simulink model "NonLinearModel"  (R2018a)
settings: Solver=VariableStepAuto  StartTime=0.0  StopTime=10  RelTol=1e-3
undefined symbols (not defined in the file): netThrust, tspan, x0
libraries: simulink x3, dspindex x3
settings Model: Creator=ojack123  LastModifiedBy=ojack123
settings OptimizationCC: DefaultParameterBehavior=Inlined  BufferReuse=off
settings DebuggingCC: InitInArrayFormatMsg=none

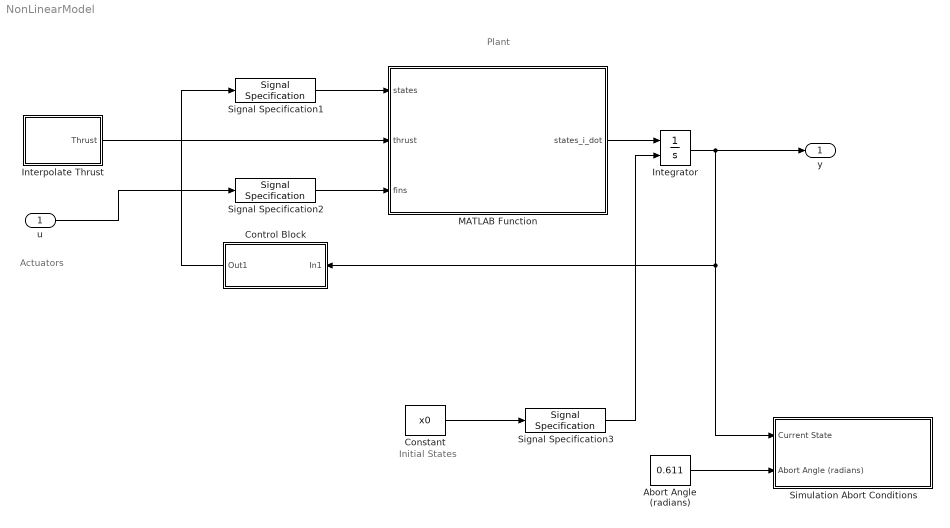
== system NonLinearModel ==
  note: Actuators
  note: Plant
  note: Initial States
  u : Inport
  Abort Angle (radians) : Constant  Value=0.611
  Constant : Constant  Value=x0
  Control Block : Subsystem
  Integrator : Integrator  InitialConditionSource=external  InitialCondition="[0 0 0 0 0 0.5 0 0    0.049979      0.99875 0.0 0.0 0]"
  Interpolate Thrust : Subsystem
  MATLAB Function : MATLAB Function  TreatAsAtomicUnit=on
  Signal Specification1 : SignalSpecification  Dimensions=[13 1]
  Signal Specification2 : SignalSpecification  Dimensions=[4 1]
  Signal Specification3 : SignalSpecification  Dimensions=[13 1]
  Simulation Abort Conditions : Subsystem
  y : Outport
  wires:
  MATLAB Function/1(states_i_dot) -> Integrator/1
  Interpolate Thrust/1(Thrust) -> MATLAB Function/2(thrust)
  Constant/1 -> Signal Specification3/1
  Integrator/1 -> y/1, Control Block/1(In1), Simulation Abort Conditions/1(Current State)
  Abort Angle (radians)/1 -> Simulation Abort Conditions/2(Abort Angle (radians))
  u/1 -> Signal Specification2/1
  Signal Specification1/1 -> MATLAB Function/1(states)
  Signal Specification2/1 -> MATLAB Function/3(fins)
  Signal Specification3/1 -> Integrator/2
  Control Block/1(Out1) -> Signal Specification1/1

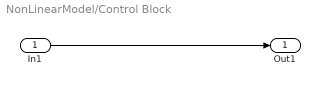
== system NonLinearModel/Control Block ==
  In1 : Inport
  Out1 : Outport
  wires:
  In1/1 -> Out1/1

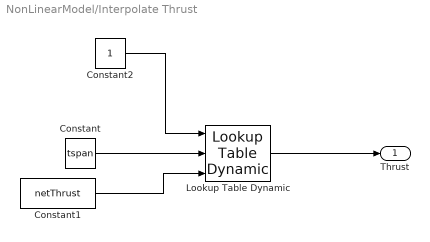
== system NonLinearModel/Interpolate Thrust ==
  Constant : Constant  Value=tspan  VectorParams1D=off
  Constant1 : Constant  Value=netThrust  VectorParams1D=off
  Constant2 : Constant
  Lookup Table Dynamic : simulink/Lookup Tables/Lookup Table Dynamic  LookUpMeth=Interpolation-Use End Values  OutDataType=fixdt('double')  OutScaling=2^-10  OutDataTypeStr=Inherit: Inherit via back propagation  RndMeth=Nearest  DoSatur=off
      settings: SourceProductName=Simulink
  Thrust : Outport
  wires:
  Constant2/1 -> Lookup Table Dynamic/1
  Lookup Table Dynamic/1 -> Thrust/1
  Constant/1 -> Lookup Table Dynamic/2
  Constant1/1 -> Lookup Table Dynamic/3

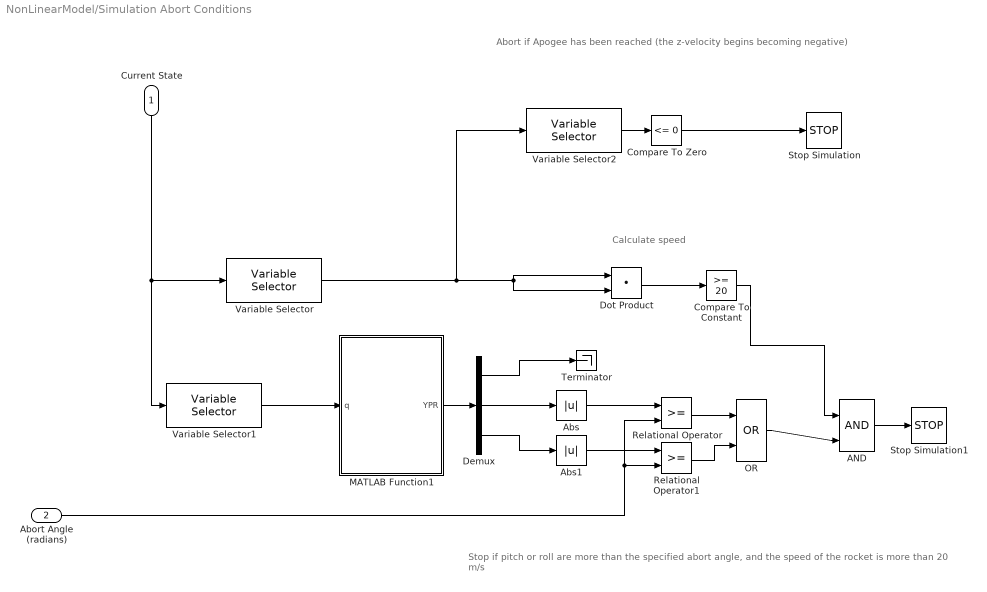
== system NonLinearModel/Simulation Abort Conditions ==
  note: Stop if pitch or roll are more than the specified abort angle, and the speed of the rocket is more than 20 m/s
  note: Calculate speed
  note: Abort if Apogee has been reached (the z-velocity begins becoming negative)
  Current State : Inport
  Abort Angle (radians) : Inport  Port=2
  AND : Logic  IconShape=distinctive  AllPortsSameDT=off  OutDataTypeStr=boolean
  Abs : Abs
  Abs1 : Abs
  Compare To Constant : simulink/Logic and Bit Operations/Compare To Constant  relop=>=  const=20  OutDataTypeStr=boolean
  Compare To Zero : simulink/Logic and Bit Operations/Compare To Zero  relop=<=  OutDataTypeStr=boolean
  Demux : Demux  Outputs=3
  Dot Product : DotProduct  InputSameDT=on  OutDataTypeStr=Inherit: Inherit via internal rule
  MATLAB Function1 : MATLAB Function  TreatAsAtomicUnit=on
  OR : Logic  Operator=OR  IconShape=distinctive  AllPortsSameDT=off  OutDataTypeStr=boolean
  Relational Operator : RelationalOperator  OutDataTypeStr=boolean  RndMeth=Simplest
  Relational Operator1 : RelationalOperator  OutDataTypeStr=boolean  RndMeth=Simplest
  Stop Simulation : Stop
  Stop Simulation1 : Stop
  Terminator : Terminator
  Variable Selector : dspindex/Variable Selector  NumInputs=1  rowsOrCols=Rows  IdxMode=Fixed  Elements=[4 5 6]  ZerOneIdxMode=One-based  errmode=Clip Index  FillMode=on  FillValues=0
  Variable Selector1 : dspindex/Variable Selector  NumInputs=1  rowsOrCols=Rows  IdxMode=Fixed  Elements=[7 8 9 10]  ZerOneIdxMode=One-based  errmode=Clip Index  FillMode=on  FillValues=0
  Variable Selector2 : dspindex/Variable Selector  NumInputs=1  rowsOrCols=Rows  IdxMode=Fixed  Elements=3  ZerOneIdxMode=One-based  errmode=Clip Index  FillMode=on  FillValues=0
  wires:
  Variable Selector/1 -> Dot Product/1, Dot Product/2, Variable Selector2/1
  OR/1 -> AND/2
  Compare To Zero/1 -> Stop Simulation/1
  Current State/1 -> Variable Selector/1, Variable Selector1/1
  Relational Operator/1 -> OR/1
  Relational Operator1/1 -> OR/2
  Variable Selector2/1 -> Compare To Zero/1
  Abort Angle (radians)/1 -> Relational Operator/2, Relational Operator1/2
  Abs1/1 -> Relational Operator1/1
  Abs/1 -> Relational Operator/1
  Compare To Constant/1 -> AND/1
  AND/1 -> Stop Simulation1/1
  Dot Product/1 -> Compare To Constant/1
  Variable Selector1/1 -> MATLAB Function1/1(q)
  Demux/2 -> Abs/1
  Demux/3 -> Abs1/1
  Demux/1 -> Terminator/1
  MATLAB Function1/1(YPR) -> Demux/1

== matlab function NonLinearModel/Simulation Abort Conditions/MATLAB Function1 ==
  data: q input; YPR output
function YPR = euler_from_q(q)
y = 0;
p = 0;
r = 0;
YPR = dcm_to_euler(dcm_from_q(q));

end
% ~~~~~~~~~~~~~~~~~~~~~~~~~~~~~~~~~~~~~~~~~~~~~~
function Q = dcm_from_q(q)
% ~~~~~~~~~~~~~~~~~~~~~~~
%{
  This function calculates the direction cosine matrix
  from the quaternion.

  q - quaternion (where q(4) is the scalar part)
  Q - direction cosine matrix
%}
% ----------------------------------------------
Q  = zeros(3);
q1 = 0;
q2 = 0;
q3 = 0;
q4 = 0;
q1 = q(1); q2 = q(2); q3 = q(3); q4 = q(4);

Q = [q1^2-q2^2-q3^2+q4^2,      2*(q1*q2+q3*q4),       2*(q1*q3-q2*q4);
         2*(q1*q2-q3*q4), -q1^2+q2^2-q3^2+q4^2,       2*(q2*q3+q1*q4);
         2*(q1*q3+q2*q4),      2*(q2*q3-q1*q4),  -q1^2-q2^2+q3^2+q4^2 ];
end %dcm_from_q
% ~~~~~~~~~~~~~~~~~~~~~~~~~~~~~~~~~~~~~~~~~~~~~~

% ~~~~~~~~~~~~~~~~~~~~~~~~~~~~~~~~~~~~~~~~~~~~~~~
function ABG = dcm_to_euler(Q)
% ~~~~~~~~~~~~~~~~~~~~~~~~~~~~~~~~~~~~~~~~~~~
%{
  This function finds the angles of the classical Euler sequence
  R3(gamma)*R1(beta)*R3(alpha) from the direction cosine matrix

  Q     - direction cosine matrix
  alpha - first angle of the sequence (deg)
  beta  - second angle of the sequence (deg)
  gamma - third angle of the sequence (deg)

  User M-function required: atan2d_0_360
%}
% -----------------------------------------------
alpha = 0;
beta  = 0;
gamma = 0;
alpha = atan2_0_360(Q(3,1), -Q(3,2));
beta  = acos(Q(3,3));
gamma = atan2_0_360(Q(1,3), Q(2,3));
ABG = [alpha beta gamma];

end
% ~~~~~~~~~~~~~~~~~~~~~~~~~~~~~~~~~~~~~~~~~~~~~~~


% ~~~~~~~~~~~~~~~~~~~~~~~~~~~~~~~~~~~~~~~~~~~~~~
function out = atan2_0_360(y,x)
% ~~~~~~~~~~~~~~~~~~~~~~~~~~~~
%{
  This function calculates the arc tangent of y/x in degrees
  and places the result in the range [0, 360].

  t - angle in degrees

%}
% ----------------------------------------------
y = 0;
x = 0;
t = 0;
out = 0;
y = rad2deg(y);
x = rad2deg(x);

if x == 0
    if y == 0
        t = 0;
    elseif y > 0
        t = 90;
    else
        t = 270;
    end    
elseif x > 0
    if y >= 0
        t = atand(y/x);
    else
        t = atand(y/x) + 360;
    end    
elseif x < 0   
    if y == 0
        t = 180;
    else
        t = atand(y/x) + 180;
    end       
end
out = deg2rad(t);
end

% ~~~~~~~~~~~~~~~~~~~~~~~~~~~~~~~~~~~~~~~~~~~~~~

== matlab function NonLinearModel/MATLAB Function ==
  data: states input; states_i_dot output; thrust input; fins input
function states_i_dot = EquationsOfMotion(states,thrust,fins)
   rocketStruct = load('rocket');
%% Define the quaternions 
    q           = states(7:10);
%% External Forces (inertial frame)
% Aerodynamic forces due to rocket body
    vel_i       = states(4:6);
    vel_b       = quaternion_I_to_B(q,vel_i);
    speed       = norm(vel_i);
    alpha       = atan2(vel_b(1),vel_b(3));
    beta        = asin(vel_b(2)/speed);
    Cx_v        = rocketStruct.rocket.Cla * (alpha);
    Cy_v        = rocketStruct.rocket.Clb * (beta);
    Cz_v        = 0.05*rocketStruct.rocket.Cd0; % Estimating the drag to be directly opposite the nose
    C_v         = [-Cx_v; -Cy_v; -Cz_v];
    Fad_v       = 0.5*(1.225)*rocketStruct.rocket.area*(speed^2).*C_v;
    Rvel2body   = (R2(-alpha)*R3(beta))';
    Fad_b       = Rvel2body *Fad_v;
Fad_i       = quaternion_B_to_I(q,Fad_b);
    
Fg_i        = [0;0;-9.8*rocketStruct.rocket.m];
    
Fexternal_i = Fg_i +Fad_i;
%% Thrust force
   thrust_b = [0;0;thrust];
netThrust_i = quaternion_B_to_I(q,thrust_b); 
    
%% Net Force on the rocket body
Fnet_i      = Fexternal_i + netThrust_i;

%% External Moments (inertial frame)
% Rotate the distance from CP to CG into the inertial frame
    cp2cg_b     = rocketStruct.rocket.dcg-rocketStruct.rocket.dcp;
    cp2cg_i     = quaternion_B_to_I(q,cp2cg_b); % distance from the cp to cg in inertial frame
% Moment due to aerodynamic force of rocket body
Mad_i       = cross(cp2cg_i,Fad_i);
% Net External Moments
Mexternal_i = Mad_i;
    
%% Moments due to Fins
% Fin locations (body fixed)
    finLatOffset = 0.1; % Flipper offset from z-axis
    finCGOffset  = -rocketStruct.rocket.dcg(3); % Flipper offset from the CG
    r1_b         = [finLatOffset;  0;            finCGOffset];
    r2_b         = [0;             finLatOffset; finCGOffset];
    r3_b         = [-finLatOffset; 0;            finCGOffset];
    r4_b         = [0;            -finLatOffset; finCGOffset];
% Fin forces
    F1_b         = [0       ; fins(1) ;0];
    F2_b         = [-fins(2); 0       ;0];
    F3_b         = [0       ; -fins(3);0];
    F4_b         = [fins(4) ; 0       ;0];
% body-fixed moments due to the flippers
    M1_b         = cross(r1_b,F1_b);
    M2_b         = cross(r2_b,F2_b);
    M3_b         = cross(r3_b,F3_b);
    M4_b         = cross(r4_b,F4_b);
    Mfins_b      = M1_b + M2_b + M3_b + M4_b;
% intertial-frame moments due to the flippers
Mfins_i      = quaternion_B_to_I(q,Mfins_b);
    
%% Net moments on the rocket body
    Mnet_i       = Mexternal_i + Mfins_i;
    Mnet_b       = quaternion_I_to_B(q,Mnet_i);
    xyz_b        = quaternion_I_to_B(q,states(11:13));
%% Omega Matrix and angular momentum to calculate qdot
    Omega       = [[0            states(13) -states(12) states(11)];
                   [-states(13)  0           states(11) states(12)];
                   [ states(12) -states(11)  0          states(13)];
                   [-states(11) -states(12) -states(13) 0         ]];
    H           =  (rocketStruct.rocket.I)'.*states(11:13);                   % angular momentum

%% Define states_i_dot as the solutions to the equations of motion
posdot_i    = states(4:6);               % inertial frame velocity
veldot_i    = Fnet_i / rocketStruct.rocket.m;         % inertial frame acceleration
q_shifted   = circshift(q,-1);           % need to move the scalar part back to the 4th index
qdot        = circshift(0.5*Omega*q_shifted,1);   % time derivative of quaternions
wdot        = ((Mnet_b-cross(states(11:13),H))' ./ (rocketStruct.rocket.I))'; % angular acceleration

%% Output term (dx)
states_i_dot    = [posdot_i; veldot_i; qdot; wdot];

%%
%%
%%
%%
%%
%%
%% Define all functions present here
%% ----------------------------------------------------------------
function B = quaternion_I_to_B(q,A)
% Rotation from Body fixed to Inertial frame
% QiB = dcm_from_q(circshift(q,-1)); %%%% Uncomment if not using Aerospace
% B = QiB*A;                         %%%% Toolbox. Delete circshift too
B = quatrotate(q',A')';
end
function I = quaternion_B_to_I(q,A)
% Rotation from Body fixed to Inertial frame
% QbI = dcm_from_q(circshift(q,-1)); %%%% Uncomment if not using Aerospace
% I = QbI'*A  ;                      %%%% Toolbox. Delete circshift too
I = quatrotate(quatconj(q'),A')';
end
function qout = quatrotate( q, r )
%  QUATROTATE Rotate a vector by a quaternion.
%   N = QUATROTATE( Q, R ) calculates the rotated vector, N, for a
%   quaternion, Q, and a vector, R.  Q is either a M-by-4 matrix
%   containing M quaternions or a single 1-by4 quaternion.  R
%   is either a M-by-3 matrix or a single 1-by-3 vector.  N returns an
%   M-by-3 matrix of rotated vectors.  Each element of Q and R must be a
%   real number.  Additionally, Q has its scalar number as the first column.
%
%   Examples:
%
%      q = [1 0 1 0];
%      r = [1 1 1];
%      n = quatrotate( q, r ) 
%
%      q = [1 0 1 0; 1 0.5 0.3 0.1];
%      r = [1 1 1];
%      n = quatrotate( q, r ) 
%
%      q = [1 0 1 0];
%      r = [1 1 1; 2 3 4];
%      n = quatrotate( q, r ) 
%
%      q = [1 0 1 0; 1 0.5 0.3 0.1];
%      r = [1 1 1; 2 3 4];
%      n = quatrotate( q, r ) 
%
%   See also QUAT2DCM, QUATCONJ, QUATDIVIDE, QUATINV, QUATMOD,
%   QUATMULTIPLY, QUATNORM, QUATNORMALIZE.

%   Copyright 2000-2010 The MathWorks, Inc.
    

dcm = quat2dcm(q);
qout = [0 0 0 0];
if ( size(q,1) == 1 ) 
    % Q is 1-by-4
    qout = (dcm*r')';
elseif (size(r,1) == 1) 
    % R is 1-by-3
    for i = size(q,1):-1:1
        qout(i,:) = (dcm(:,:,i)*r')';
    end
else
    % Q is M-by-4 and R is M-by-3
    for i = size(q,1):-1:1
        qout(i,:) = (dcm(:,:,i)*r(i,:)')';
    end
end
end
function dcm = quat2dcm( q )
%  QUAT2DCM Convert quaternion to direction cosine matrix.
%   N = QUAT2DCM( Q ) calculates the direction cosine matrix, N, for a
%   given quaternion, Q.  Input Q is an M-by-4 matrix containing M
%   quaternions.  N returns a 3-by-3-by-M matrix of direction cosine 
%   matrices.  The direction cosine matrix performs the coordinate
%   transformation of a vector in inertial axes to a vector in body axes.
%   Each element of Q must be a real number.  Additionally, Q has its
%   scalar number as the first column. 
%
%   Examples:
%
%   Determine the direction cosine matrix from q = [1 0 1 0]:
%      dcm = quat2dcm([1 0 1 0])
%
%   Determine the direction cosine matrices from multiple quaternions:
%      q = [1 0 1 0; 1 0.5 0.3 0.1];
%      dcm = quat2dcm(q)
%
%   See also ANGLE2DCM, DCM2ANGLE, DCM2QUAT, ANGLE2QUAT, QUAT2ANGLE, QUATROTATE. 

%   Copyright 2000-2007 The MathWorks, Inc.
qin = [0 0 0 0];
qin = quatnormalize( q );

dcm = zeros(3,3,size(qin,1));

dcm(1,1,:) = qin(:,1).^2 + qin(:,2).^2 - qin(:,3).^2 - qin(:,4).^2;
dcm(1,2,:) = 2.*(qin(:,2).*qin(:,3) + qin(:,1).*qin(:,4));
dcm(1,3,:) = 2.*(qin(:,2).*qin(:,4) - qin(:,1).*qin(:,3));
dcm(2,1,:) = 2.*(qin(:,2).*qin(:,3) - qin(:,1).*qin(:,4));
dcm(2,2,:) = qin(:,1).^2 - qin(:,2).^2 + qin(:,3).^2 - qin(:,4).^2;
dcm(2,3,:) = 2.*(qin(:,3).*qin(:,4) + qin(:,1).*qin(:,2));
dcm(3,1,:) = 2.*(qin(:,2).*qin(:,4) + qin(:,1).*qin(:,3));
dcm(3,2,:) = 2.*(qin(:,3).*qin(:,4) - qin(:,1).*qin(:,2));
dcm(3,3,:) = qin(:,1).^2 - qin(:,2).^2 - qin(:,3).^2 + qin(:,4).^2;
end
function qout = quatnormalize( q )
%  QUATNORMALIZE Normalize a quaternion.
%   N = QUATNORMALIZE( Q ) calculates the normalized quaternion, N, for a
%   given quaternion, Q.  Input Q is an M-by-4 matrix containing M
%   quaternions.  N returns an M-by-4 matrix of normalized quaternions.
%   Each element of Q must be a real number.  Additionally, Q has its
%   scalar number as the first column.
%
%   Examples:
%
%   Normalize q = [1 0 1 0]:
%      normal = quatnormalize([1 0 1 0])
%
%   See also QUATCONJ, QUATDIVIDE, QUATINV, QUATMOD, QUATMULTIPLY, 
%   QUATNORM, QUATROTATE.

%   Copyright 2000-2005 The MathWorks, Inc.

qout = q./(quatmod( q )* ones(1,4));
end
function mod = quatmod( q )
%  QUATMOD Calculate the modulus of a quaternion.
%   N = QUATMOD( Q ) calculates the modulus, N, for a given quaternion, Q.  
%   Input Q is an M-by-4 matrix containing M quaternions.  N returns a 
%   column vector of M moduli.  Each element of Q must be a real number.  
%   Additionally, Q has its scalar number as the first column.
%
%   Examples:
%
%   Determine the modulus of q = [1 0 0 0]:
%      mod = quatmod([1 0 0 0])
%
%   See also QUATCONJ, QUATDIVIDE, QUATINV, QUATMULTIPLY, QUATNORM,
%   QUATNORMALIZE, QUATROTATE.

%   Copyright 2000-2017 The MathWorks, Inc.


mod = sqrt(quatnorm(q));
end
function qout = quatnorm( q )
%  QUATNORM Calculate the norm of a quaternion.
%   N = QUATNORM( Q ) calculates the norm, N, for a given quaternion, Q.  Input
%   Q is an M-by-4 matrix containing M quaternions.  N returns a column vector
%   of M norms.  Each element of Q must be a real number.  Additionally, Q has
%   its scalar number as the first column.
%
%   Examples:
%
%   Determine the norm of q = [1 0 0 0]:
%      norm = quatnorm([1 0 0 0])
%
%   See also QUATCONJ, QUATDIVIDE, QUATINV, QUATMOD, QUATMULTIPLY, 
%   QUATNORMALIZE, QUATROTATE.

%   Copyright 2000-2017 The MathWorks, Inc.
qout = [0 0 0 0];
qout = sum(q.^2,2);

end
function qout = quatconj( qin ) 
%  QUATCONJ Calculate the conjugate of a quaternion.
%   N = QUATCONJ( Q ) calculates the conjugate, N, for a given quaternion, Q.  
%   Input Q is an M-by-4 matrix containing M quaternions.  N returns an 
%   M-by-4 matrix of conjugates.  Each element of Q must be a real number.  
%   Additionally, Q has its scalar number as the first column.
%
%   Examples:
%
%   Determine the conjugate of q = [1 0 1 0]:
%      conj = quatconj([1 0 1 0])
%
%   See also QUATDIVIDE, QUATINV, QUATMOD, QUATMULTIPLY, QUATNORM, 
%   QUATNORMALIZE, QUATROTATE.

%   Copyright 2000-2010 The MathWorks, Inc.
qout = [0 0 0 0];
qout = [ qin(:,1)  -qin(:,2:4) ];
end
end
